simulink model "sampleModel1818_3_sub_sub"  (R2023a)
settings: Solver=VariableStepAuto  StartTime=0.0  StopTime=10.0  RelTol=1e-3
libraries: simulink x3, hdlsllib x3
settings Model: Creator=user1  LastModifiedBy=user1

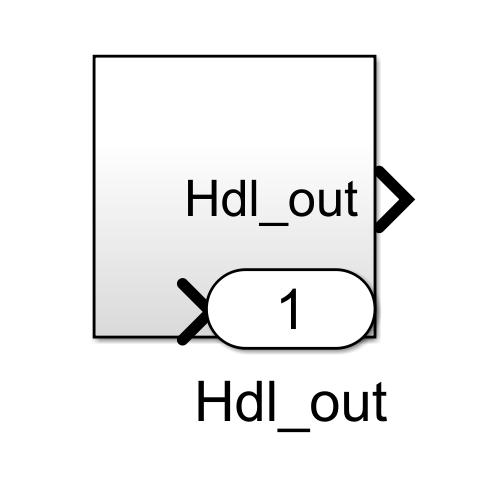
[thumbnail: Simulink's stored preview of the top-level diagram]
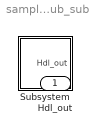
== system sampleModel1818_3_sub_sub ==
  Subsystem : Subsystem
  Hdl_out : Outport  OutDataTypeStr=uint8

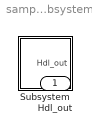
== system sampleModel1818_3_sub_sub/Subsystem ==
  Subsystem : Subsystem
  Hdl_out : Outport  OutDataTypeStr=uint8

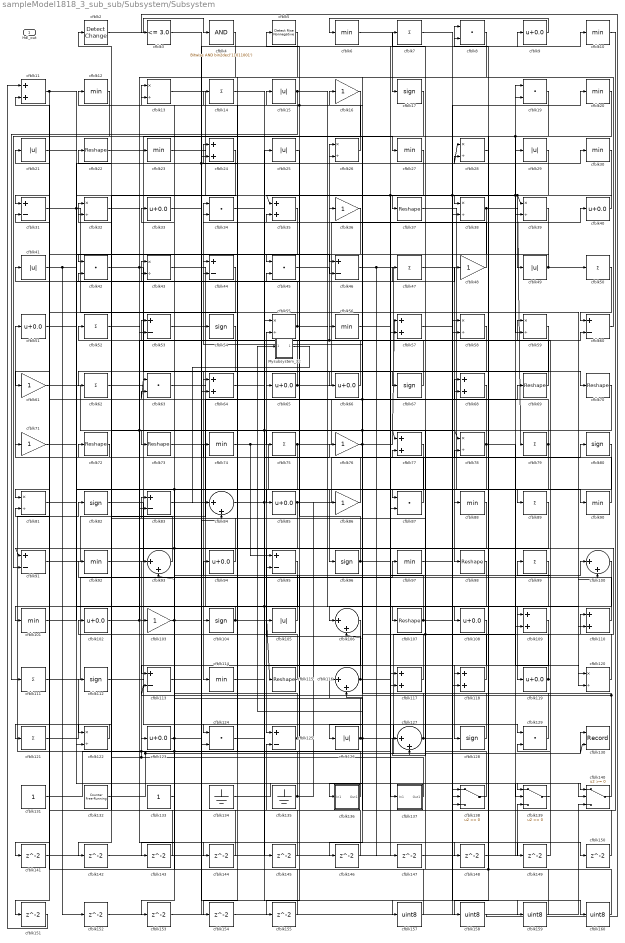
== system sampleModel1818_3_sub_sub/Subsystem/Subsystem ==
  Mysubsystem_32 : Subsystem  TreatAsAtomicUnit=on  RTWFcnName=Mysubsystem_32
      settings: RTWFcnNameOpts=User specified  RTWFileNameOpts=Use function name
  cfblk{6,10,12,20,23,27,30,56,74,88,90,92,97,101,114} (15 alike) : MinMax  OutDataTypeStr=uint8
  cfblk{84,93,100,106,116,127} (6 alike) : Sum  Inputs=|++  OutDataTypeStr=uint8
  cfblk{9,33,40,51,65..66,85,94,102,108,119,123} (12 alike) : Bias  Bias=0.0  SaturateOnIntegerOverflow=off
  cfblk{16,36,48,61,71,76,86,103} (8 alike) : Gain  OutDataTypeStr=uint8
  cfblk{17,54,67,80,82,96,104,112,128} (9 alike) : Signum
  cfblk{15,21,25,29,41,49,105,126} (8 alike) : Abs  OutDataTypeStr=uint8  SaturateOnIntegerOverflow=off
  cfblk{22,37,69..70,72..73,98,107,115} (9 alike) : Reshape
  cfblk{11,24,35,57,64,68,77,109..110,117..118} (11 alike) : Sum  OutDataTypeStr=uint8
  cfblk{7,14,47,50,52,62,75,79,89,99,111,121} (12 alike) : Sum  Inputs=+  OutDataTypeStr=uint8
  cfblk{31,44,46,53,60,83,91,95,113,125} (10 alike) : Sum  Inputs=+-  OutDataTypeStr=uint8
  cfblk{13,26,28,32,38..39,43,55,58..59,78,81,120,122} (14 alike) : Product  Inputs=*/  OutDataTypeStr=uint8  RndMeth=Zero  SaturateOnIntegerOverflow=on
  cfblk{8,19,34,42,45,63,87,124,129} (9 alike) : DotProduct  OutDataTypeStr=uint8
  cfblk130 : Record  FileSettingsInternal="{\"entries\":[{\"content\":{\"excelSettings\":{\"content\":{},\"type\":\"Streamout.ExcelSettings\"}},\"type\":\"Streamout.FileSettingStorage\",\"uuid\":\"\"}],\"packageUris\":[\"http:\\/\\/schema.mathworks.com\\/mf0\\/streamout_blocks\\/R2020a\"],\"version\":\"1.0\"}"  Layout=[1 1]  SignalsInternal="{\"entries\":[{\"content\":{\"signals\":[{\"content\":{\"blockPath\":[],\"dimensions\":[1],\"domain\":\"\",\"lineColor\":\"#a2142f\",\"plots\":[1],\"port\":1,\"signalID\":43251,\"signalName\":\"cfblk112\"},\"type\":\"RecordBlkView.Signal\",\"uuid\":\"\"},{\"content\":{\"blockPath\":[],\"dimensions\":[1],\"domain\":\"\",\"lineColor\":\"#139fff\",\"plots\":[1],\"port\":2,\"signalID\":43254,\"signalName\":\"cfblk132\"},\"type\":\"RecordBlkView.Signal\",\"uuid\":\"\"}]},\"type\":\"RecordBlkView.InputSignals\",\"uuid\":\"\"}],\"packageUris\":[\"http:\\/\\/schema.mathworks.com\\/mf0\\/streamout_blocks\\/R2020a\"],\"version\":\"1.0\"}"  VisualizationBindings="{\"xyplotplugin\":{\"info\":[{\"series\":[{\"bindingParametersList\":[{\"parameter\":\"X-Axis\",\"signalID\":43251,\"signalName\":\"cfblk112\"},{\"parameter\":\"Y-Axis\",\"signalID\":43254,\"signalName\":\"cfblk132\"}],\"seriesID\":46672}],\"subplotID\":1}]}}"  CompatibilityTag=XY  st=-1
  cfblk131 : Constant  OutDataTypeStr=uint8  SampleTime=-1
  cfblk132 : hdlsllib/Sources/Counter Free-Running  NumBits=16  tsamp=-1
  cfblk133 : Constant  OutDataTypeStr=uint8  SampleTime=-1
  cfblk134 : Ground
  cfblk135 : Ground
  cfblk136 : Subsystem
      settings: LibrarySourceBlock=|
      | hdlsllib/Ports &
      | Subsystems/Subsystem
  cfblk137 : Subsystem
      settings: LibrarySourceBlock=|
      | hdlsllib/Ports &
      | Subsystems/Subsystem
  cfblk138 : Switch  OutDataTypeStr=uint8  SaturateOnIntegerOverflow=off  InputSameDT=off
  cfblk139 : Switch  OutDataTypeStr=uint8  SaturateOnIntegerOverflow=off  InputSameDT=off
  cfblk140 : Switch  OutDataTypeStr=uint8  SaturateOnIntegerOverflow=off  InputSameDT=off
  cfblk{141..155} (15 alike) : Delay  SampleTime=1
  cfblk{157..160} (4 alike) : DataTypeConversion  OutDataTypeStr=uint8  SaturateOnIntegerOverflow=off  RndMeth=Floor
  cfblk2 : simulink/Logic and Bit Operations/Detect Change  vinit=0  OutDataTypeStr=uint8
      settings: LibrarySourceBlock=|
      | hdlsllib/Logic and Bit
      | Operations/Detect
      | Change
  cfblk3 : hdlsllib/Logic and Bit Operations/Compare To Constant  relop=<=  const=3.0  OutDataTypeStr=uint8
  cfblk4 : simulink/Logic and Bit Operations/Bitwise Operator  logicop=AND  UseBitMask=on  BitMask=bin2dec('11011001')  BitMaskRealWorld=Stored Integer
      settings: LibrarySourceBlock=|
      | hdlsllib/Logic and Bit
      | Operations/Bitwise
      | Operator
  cfblk5 : hdlsllib/Logic and Bit Operations/Detect Rise Nonnegative  vinit=0  OutDataTypeStr=uint8
  Hdl_out : Outport  OutDataTypeStr=uint8
  wires:
  Mysubsystem_32/1(Out1) -> cfblk84/1
  cfblk160/1 -> cfblk7/1
  cfblk124/1 -> cfblk160/1
  cfblk159/1 -> cfblk8/2, cfblk71/1
  cfblk158/1 -> cfblk3/1
  cfblk157/1 -> cfblk21/1
  cfblk3/1 -> cfblk157/1
  cfblk155/1 -> cfblk43/2
  cfblk39/1 -> cfblk155/1
  cfblk154/1 -> cfblk58/1
  cfblk8/1 -> cfblk154/1
  cfblk153/1 -> cfblk84/2
  cfblk152/1 -> cfblk140/3
  cfblk151/1 -> cfblk11/1
  cfblk16/1 -> cfblk151/1
  cfblk150/1 -> cfblk116/1
  cfblk149/1 -> cfblk129/2
  cfblk148/1 -> cfblk19/1
  cfblk147/1 -> cfblk139/3
  cfblk146/1 -> cfblk81/2
  cfblk80/1 -> cfblk146/1
  cfblk145/1 -> cfblk125/2
  cfblk34/1 -> cfblk145/1
  cfblk144/1 -> cfblk31/2
  cfblk143/1 -> cfblk42/2
  cfblk142/1 -> cfblk57/2
  cfblk24/1 -> cfblk142/1
  cfblk141/1 -> cfblk55/1
  cfblk44/1 -> cfblk141/1
  cfblk56/1 -> cfblk9/1
  cfblk117/1 -> cfblk34/2, cfblk63/1
  cfblk105/1 -> cfblk43/1
  cfblk52/1 -> cfblk77/1, cfblk144/1
  cfblk54/1 -> cfblk64/2
  cfblk11/1 -> cfblk31/1, cfblk109/1
  cfblk137/1(Out1) -> cfblk123/1, cfblk32/2
  cfblk93/1 -> cfblk12/1
  cfblk133/1 -> cfblk103/1
  cfblk51/1 -> cfblk47/1
  cfblk45/1 -> cfblk46/2
  cfblk139/1 -> cfblk99/1
  cfblk101/1 -> cfblk28/2
  cfblk134/1 -> cfblk139/2
  cfblk5/1 -> cfblk53/2
  cfblk4/1 -> cfblk24/2
  cfblk129/1 -> cfblk54/1
  cfblk19/1 -> cfblk116/2, cfblk39/2
  cfblk84/1 -> cfblk118/2, cfblk109/2, cfblk76/1
  cfblk107/1 -> cfblk94/1, cfblk149/1
  cfblk70/1 -> cfblk127/2
  cfblk89/1 -> cfblk117/2
  cfblk14/1 -> cfblk140/1, cfblk78/1
  cfblk53/1 -> cfblk44/2
  cfblk57/1 -> cfblk139/1
  cfblk103/1 -> cfblk53/1, cfblk108/1
  cfblk128/1 -> cfblk13/1
  cfblk75/1 -> cfblk58/2, cfblk122/2
  cfblk140/1 -> cfblk113/2, cfblk78/2
  cfblk132/1 -> cfblk130/2, cfblk8/1
  cfblk28/1 -> cfblk118/1
  cfblk97/1 -> cfblk20/1
  cfblk10/1 -> cfblk127/1
  cfblk30/1 -> cfblk49/1, cfblk136/1(In1)
  cfblk87/1 -> cfblk74/1
  cfblk83/1 -> cfblk117/1
  cfblk126/1 -> Mysubsystem_32/1(In1), cfblk19/2, cfblk13/2
  cfblk73/1 -> cfblk65/1
  cfblk138/1 -> cfblk83/1
  cfblk6/1 -> cfblk17/1
  cfblk38/1 -> cfblk79/1, cfblk124/2
  cfblk106/1 -> cfblk113/1
  cfblk71/1 -> cfblk88/1
  cfblk96/1 -> cfblk45/2, cfblk69/1
  cfblk131/1 -> cfblk93/1, cfblk48/1
  cfblk114/1 -> cfblk129/1
  cfblk9/1 -> cfblk6/1
  cfblk120/1 -> cfblk68/2
  cfblk41/1 -> cfblk46/1, cfblk152/1
  cfblk119/1 -> cfblk92/1, cfblk59/1
  cfblk78/1 -> cfblk83/2, cfblk143/1, cfblk75/1, cfblk120/2
  cfblk55/1 -> cfblk11/2, cfblk90/1
  cfblk109/1 -> cfblk138/3
  cfblk118/1 -> cfblk72/1, cfblk77/2
  cfblk23/1 -> cfblk137/1(In1)
  cfblk26/1 -> cfblk5/1, cfblk2/1
  cfblk99/1 -> cfblk119/1
  cfblk66/1 -> cfblk15/1
  cfblk36/1 -> cfblk64/1
  cfblk63/1 -> cfblk107/1
  cfblk100/1 -> cfblk138/2
  cfblk22/1 -> cfblk23/1
  cfblk29/1 -> cfblk59/2, cfblk158/1
  cfblk32/1 -> cfblk45/1
  cfblk98/1 -> cfblk126/1
  cfblk86/1 -> cfblk35/2
  cfblk135/1 -> cfblk44/1, cfblk86/1
  cfblk48/1 -> cfblk24/1
  cfblk27/1 -> cfblk35/1, cfblk87/2
  cfblk90/1 -> cfblk36/1
  cfblk125/1 -> cfblk33/1, cfblk95/2
  cfblk21/1 -> cfblk38/2, cfblk39/1
  cfblk123/1 -> cfblk63/2, cfblk148/1
  cfblk64/1 -> cfblk25/1
  cfblk20/1 -> cfblk98/1
  cfblk25/1 -> cfblk105/1
  cfblk7/1 -> cfblk159/1
  cfblk91/1 -> cfblk68/1
  cfblk95/1 -> cfblk104/1
  cfblk81/1 -> cfblk30/1
  cfblk60/1 -> cfblk16/1
  cfblk62/1 -> cfblk67/1
  cfblk13/1 -> cfblk38/1
  cfblk49/1 -> cfblk42/1, cfblk50/1
  cfblk68/1 -> cfblk122/1, cfblk106/2
  cfblk59/1 -> cfblk62/1
  cfblk74/1 -> cfblk138/1, cfblk95/1
  cfblk79/1 -> cfblk41/1, cfblk87/1
  cfblk43/1 -> cfblk85/1
  cfblk76/1 -> cfblk57/1, cfblk106/1
  cfblk69/1 -> cfblk22/1, cfblk56/1
  cfblk40/1 -> cfblk37/1
  cfblk113/1 -> cfblk26/2
  cfblk46/1 -> cfblk70/1, cfblk147/1
  cfblk17/1 -> cfblk91/2
  cfblk102/1 -> cfblk60/2, cfblk150/1
  cfblk77/1 -> cfblk96/1
  cfblk35/1 -> cfblk81/1
  cfblk88/1 -> cfblk91/1, cfblk153/1
  cfblk58/1 -> cfblk114/1
  cfblk104/1 -> cfblk115/1, cfblk101/1
  cfblk50/1 -> cfblk60/1
  cfblk12/1 -> cfblk61/1
  cfblk31/1 -> cfblk120/1, cfblk140/2
  cfblk15/1 -> cfblk111/1, cfblk110/2
  cfblk47/1 -> cfblk110/1
  cfblk115/1 -> cfblk102/1
  cfblk82/1 -> cfblk124/1
  cfblk37/1 -> cfblk89/1
  cfblk2/1 -> cfblk4/1
  cfblk85/1 -> cfblk125/1, cfblk29/1
  cfblk42/1 -> cfblk66/1, cfblk100/2
  cfblk122/1 -> cfblk121/1
  cfblk72/1 -> cfblk51/1
  cfblk112/1 -> cfblk130/1
  cfblk108/1 -> cfblk128/1
  cfblk94/1 -> cfblk32/1
  cfblk116/1 -> cfblk55/2, cfblk100/1
  cfblk61/1 -> cfblk73/1
  cfblk121/1 -> cfblk112/1
  cfblk110/1 -> cfblk52/1
  cfblk65/1 -> cfblk40/1, cfblk14/1
  cfblk33/1 -> cfblk28/1, cfblk10/1
  cfblk136/1(Out1) -> cfblk82/1, cfblk93/2
  cfblk111/1 -> cfblk97/1
  cfblk92/1 -> cfblk27/1
  cfblk127/1 -> cfblk34/1, cfblk80/1
  cfblk67/1 -> cfblk26/1

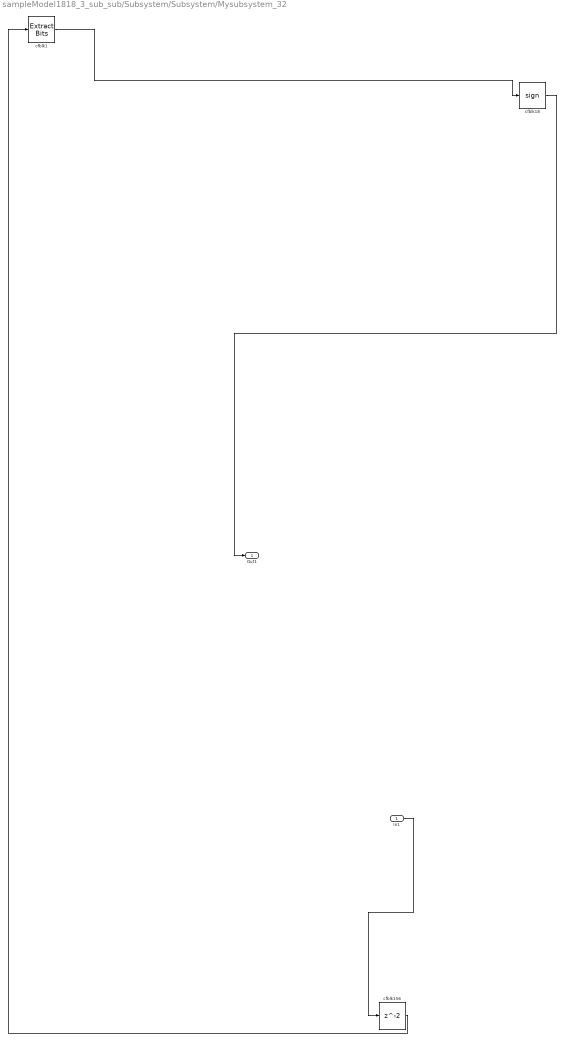
== system sampleModel1818_3_sub_sub/Subsystem/Subsystem/Mysubsystem_32 ==
  In1 : Inport
  cfblk1 : simulink/Logic and Bit Operations/Extract Bits  bitsToExtract=Upper half  numBits=8  bitIdxRange=[0 7]  outScalingMode=Preserve fixed-point scaling
      settings: LibrarySourceBlock=|
      | hdlsllib/Logic and Bit
      | Operations/Extract Bits
  cfblk156 : Delay  SampleTime=1
  cfblk18 : Signum
  Out1 : Outport
  wires:
  cfblk1/1 -> cfblk18/1
  cfblk18/1 -> Out1/1
  cfblk156/1 -> cfblk1/1
  In1/1 -> cfblk156/1

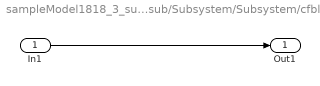
== system sampleModel1818_3_sub_sub/Subsystem/Subsystem/cfblk136 ==
  In1 : Inport
  Out1 : Outport
  wires:
  In1/1 -> Out1/1

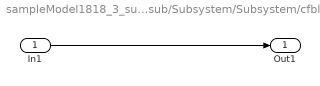
== system sampleModel1818_3_sub_sub/Subsystem/Subsystem/cfblk137 ==
  In1 : Inport
  Out1 : Outport
  wires:
  In1/1 -> Out1/1
